simulink model "gm_uz_pmsm_model_6LUT_pd"  (R2023a)
settings: Solver=FixedStepAuto  StartTime=0.0  StopTime=0.05  RelTol=1e-3
PreLoadFcn:
  | uz_pmsm_model_init_parameter
PostLoadFcn:
  | % Import the data from Excel for a lookup table
  | FluxMapData = readtable('C:\Users\Philipp\ultrazohm\ultrazohm_sw\ip_cores\uz_pmsm_model\FluxMapData_2023-05-26_13-07-57.csv');
  | % Row indices for lookup table
  | d_current_in_d_axis = FluxMapData(8:27,1:end);
  | % Column indices for lookup table
  | q_current_in_d_axis = FluxMapData(29:48,1:end);
  | % Output values for lookup table
  | d_Flux_d_axis = FluxMapData(50:69,1:end);
undefined symbols (not defined in the file or in its folder): d_current_d_Flux, d_current_q_Flux, entkopplung_dynamic, entkopplung_linear, entkopplung_static, Flux_d, Flux_q, friction_coefficient, inertia, k_i_d, k_p_d, k_p_q, Ki_Bo_d, Ki_Bo_q, Kp_Bo_d, Kp_Bo_q, L_d, L_q, Ldd, Ldq, Lqd, Lqq, parameter_nachfuerung, polepair, praediktion_entkopplung_nonlinear, psi_pm, q_current_d_Flux, q_current_q_Flux, R_1, simulate_mechanical, simulate_nonlinear_modell, simulate_open_loop, static_friction_torque, tau_sum, ts, ts_regler
libraries: hdlmdlgenlib x5, slpidlib x4
(part 2 of 2)

== system gm_uz_pmsm_model_6LUT_pd/Current_Controller/Psi_d_q ==
  I_d_set : Inport
  I_d : Inport  Port=2
  I_q_set : Inport  Port=3
  I_q : Inport  Port=4
  Flux_d Lookup Table : Lookup_n-D  BreakpointsForDimension1=d_current_d_Flux  BreakpointsForDimension2=q_current_d_Flux  BreakpointsForDimension3=[5, 7]  Table=Flux_d  InternalRulePriority=Speed  RndMeth=Simplest
      settings: InputPortMap=u0,u1
  Flux_d Lookup Table1 : Lookup_n-D  BreakpointsForDimension1=d_current_d_Flux  BreakpointsForDimension2=q_current_d_Flux  BreakpointsForDimension3=[5, 7]  Table=Flux_d  InternalRulePriority=Speed  RndMeth=Simplest
      settings: InputPortMap=u0,u1
  Flux_q Lookup Table1 : Lookup_n-D  BreakpointsForDimension1=d_current_q_Flux  BreakpointsForDimension2=q_current_q_Flux  BreakpointsForDimension3=[5, 7]  Table=Flux_q  InternalRulePriority=Speed  RndMeth=Simplest
      settings: InputPortMap=u0,u1
  Flux_q Lookup Table2 : Lookup_n-D  BreakpointsForDimension1=d_current_q_Flux  BreakpointsForDimension2=q_current_q_Flux  BreakpointsForDimension3=[5, 7]  Table=Flux_q  InternalRulePriority=Speed  RndMeth=Simplest
      settings: InputPortMap=u0,u1
  psi_d_set : Outport
  psi_q_set : Outport  Port=2
  psi_d_LUT : Outport  Port=3
  psi_q_LUT : Outport  Port=4
  wires:
  Flux_q Lookup Table1/1 -> psi_q_LUT/1  "psi_q_LUT"
  Flux_d Lookup Table/1 -> psi_d_LUT/1  "psi_d_LUT"
  Flux_q Lookup Table2/1 -> psi_q_set/1  "psi_q_set"
  Flux_d Lookup Table1/1 -> psi_d_set/1  "psi_d_set"
  I_q_set/1 -> Flux_q Lookup Table2/2
  I_d_set/1 -> Flux_d Lookup Table1/1
  I_q/1 -> Flux_d Lookup Table/2, Flux_d Lookup Table1/2, Flux_q Lookup Table1/2
  I_d/1 -> Flux_d Lookup Table/1, Flux_q Lookup Table1/1, Flux_q Lookup Table2/1

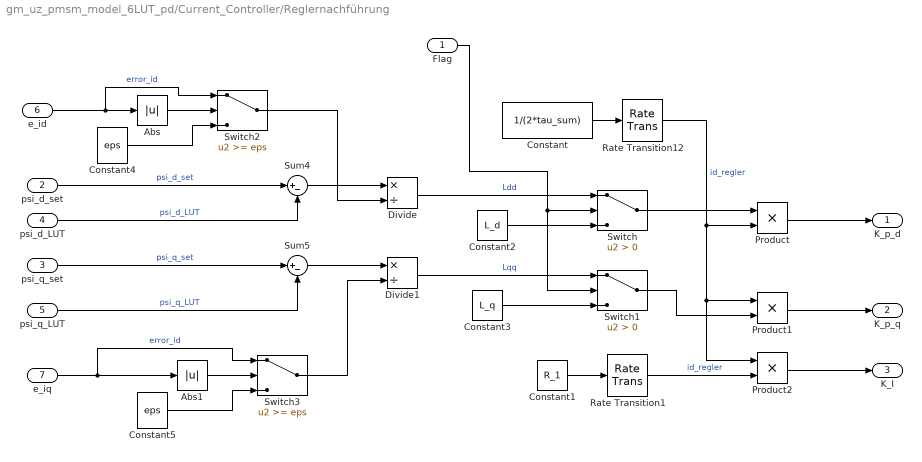
== system gm_uz_pmsm_model_6LUT_pd/Current_Controller/Reglernachführung ==
  Flag : Inport
  psi_d_set : Inport  Port=2
  psi_q_set : Inport  Port=3
  psi_d_LUT : Inport  Port=4
  psi_q_LUT : Inport  Port=5
  e_id : Inport  Port=6
  e_iq : Inport  Port=7
  Abs : Abs  SaturateOnIntegerOverflow=off
  Abs1 : Abs  SaturateOnIntegerOverflow=off
  Constant : Constant  Value=1/(2*tau_sum)
  Constant1 : Constant  Value=R_1
  Constant2 : Constant  Value=L_d
  Constant3 : Constant  Value=L_q
  Constant4 : Constant  Value=eps  SampleTime=ts_regler
  Constant5 : Constant  Value=eps  SampleTime=ts_regler
  Divide : Product  Inputs=*/
  Divide1 : Product  Inputs=*/
  Product : Product
  Product1 : Product
  Product2 : Product
  Rate Transition1 : RateTransition  OutPortSampleTime=ts_regler
  Rate Transition12 : RateTransition  OutPortSampleTime=ts_regler
  Sum4 : Sum  Inputs=|+-
  Sum5 : Sum  Inputs=|+-
  Switch : Switch  Criteria=u2 > Threshold  SaturateOnIntegerOverflow=off  InputSameDT=off
  Switch1 : Switch  Criteria=u2 > Threshold  SaturateOnIntegerOverflow=off  InputSameDT=off
  Switch2 : Switch  Threshold=eps  SaturateOnIntegerOverflow=off  InputSameDT=off
  Switch3 : Switch  Threshold=eps  SaturateOnIntegerOverflow=off  InputSameDT=off
  K_p_d : Outport
  K_p_q : Outport  Port=2
  K_I : Outport  Port=3
  wires:
  Constant5/1 -> Switch3/3
  Abs1/1 -> Switch3/2
  Switch3/1 -> Divide1/2
  e_iq/1 -> Abs1/1, Switch3/1  "error_id"
  Switch2/1 -> Divide/2
  Abs/1 -> Switch2/2
  Constant4/1 -> Switch2/3
  e_id/1 -> Abs/1, Switch2/1  "error_id"
  Divide1/1 -> Switch1/1  "Lqq"
  Divide/1 -> Switch/1  "Ldd"
  psi_q_set/1 -> Sum5/1  "psi_q_set"
  psi_d_set/1 -> Sum4/1  "psi_d_set"
  psi_d_LUT/1 -> Sum4/2  "psi_d_LUT"
  Sum5/1 -> Divide1/1
  psi_q_LUT/1 -> Sum5/2  "psi_q_LUT"
  Sum4/1 -> Divide/1
  Switch1/1 -> Product1/2
  Constant3/1 -> Switch1/3
  Switch/1 -> Product/1
  Constant2/1 -> Switch/3
  Flag/1 -> Switch1/2, Switch/2
  Rate Transition1/1 -> Product2/2  "id_regler"
  Rate Transition12/1 -> Product/2, Product1/1, Product2/1  "id_regler"
  Constant1/1 -> Rate Transition1/1
  Product2/1 -> K_I/1
  Product1/1 -> K_p_q/1
  Product/1 -> K_p_d/1
  Constant/1 -> Rate Transition12/1

== system gm_uz_pmsm_model_6LUT_pd/FOC_controller1/Psi_d_q ==
  I_d_set : Inport
  I_d : Inport  Port=2
  I_q_set : Inport  Port=3
  I_q : Inport  Port=4
  Flux_d Lookup Table : Lookup_n-D  BreakpointsForDimension1=d_current_d_Flux  BreakpointsForDimension2=q_current_d_Flux  BreakpointsForDimension3=[5, 7]  Table=Flux_d  InternalRulePriority=Speed  RndMeth=Simplest
      settings: InputPortMap=u0,u1
  Flux_d Lookup Table1 : Lookup_n-D  BreakpointsForDimension1=d_current_d_Flux  BreakpointsForDimension2=q_current_d_Flux  BreakpointsForDimension3=[5, 7]  Table=Flux_d  InternalRulePriority=Speed  RndMeth=Simplest
      settings: InputPortMap=u0,u1
  Flux_q Lookup Table1 : Lookup_n-D  BreakpointsForDimension1=d_current_q_Flux  BreakpointsForDimension2=q_current_q_Flux  BreakpointsForDimension3=[5, 7]  Table=Flux_q  InternalRulePriority=Speed  RndMeth=Simplest
      settings: InputPortMap=u0,u1
  Flux_q Lookup Table2 : Lookup_n-D  BreakpointsForDimension1=d_current_q_Flux  BreakpointsForDimension2=q_current_q_Flux  BreakpointsForDimension3=[5, 7]  Table=Flux_q  InternalRulePriority=Speed  RndMeth=Simplest
      settings: InputPortMap=u0,u1
  psi_d_set : Outport
  psi_q_set : Outport  Port=2
  psi_d_LUT : Outport  Port=3
  psi_q_LUT : Outport  Port=4
  wires:
  Flux_q Lookup Table1/1 -> psi_q_LUT/1  "psi_q_LUT"
  Flux_d Lookup Table/1 -> psi_d_LUT/1  "psi_d_LUT"
  Flux_q Lookup Table2/1 -> psi_q_set/1  "psi_q_set"
  Flux_d Lookup Table1/1 -> psi_d_set/1  "psi_d_set"
  I_q_set/1 -> Flux_q Lookup Table2/2
  I_d_set/1 -> Flux_d Lookup Table1/1
  I_q/1 -> Flux_d Lookup Table/2, Flux_d Lookup Table1/2, Flux_q Lookup Table1/2
  I_d/1 -> Flux_d Lookup Table/1, Flux_q Lookup Table1/1, Flux_q Lookup Table2/1

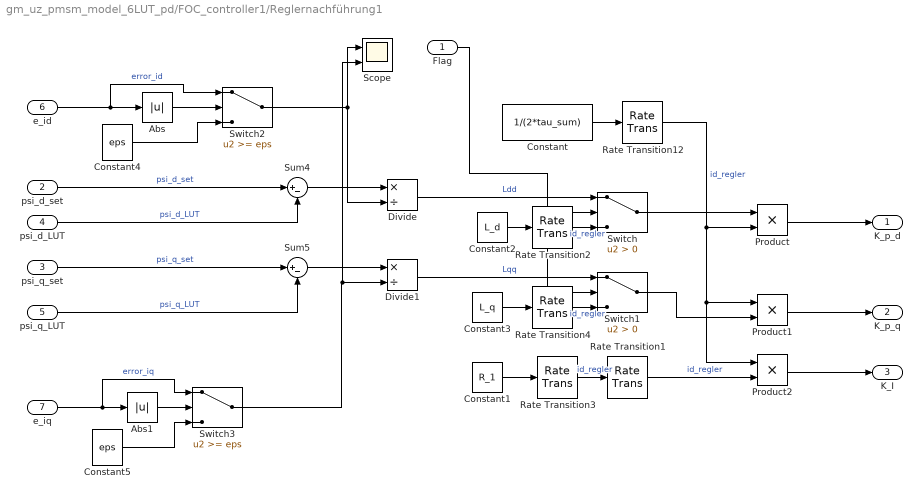
== system gm_uz_pmsm_model_6LUT_pd/FOC_controller1/Reglernachführung1 ==
  Flag : Inport
  psi_d_set : Inport  Port=2
  psi_q_set : Inport  Port=3
  psi_d_LUT : Inport  Port=4
  psi_q_LUT : Inport  Port=5
  e_id : Inport  Port=6
  e_iq : Inport  Port=7
  Abs : Abs  SaturateOnIntegerOverflow=off
  Abs1 : Abs  SaturateOnIntegerOverflow=off
  Constant : Constant  Value=1/(2*tau_sum)
  Constant1 : Constant  Value=R_1
  Constant2 : Constant  Value=L_d
  Constant3 : Constant  Value=L_q
  Constant4 : Constant  Value=eps  SampleTime=ts_regler
  Constant5 : Constant  Value=eps  SampleTime=ts_regler
  Divide : Product  Inputs=*/
  Divide1 : Product  Inputs=*/
  Product : Product
  Product1 : Product
  Product2 : Product
  Rate Transition{1..4,12} (5 alike) : RateTransition  OutPortSampleTime=ts_regler
  Scope : Scope  NumInputPorts=2
  Sum4 : Sum  Inputs=|+-
  Sum5 : Sum  Inputs=|+-
  Switch : Switch  Criteria=u2 > Threshold  SaturateOnIntegerOverflow=off  InputSameDT=off
  Switch1 : Switch  Criteria=u2 > Threshold  SaturateOnIntegerOverflow=off  InputSameDT=off
  Switch2 : Switch  Threshold=eps  SaturateOnIntegerOverflow=off  InputSameDT=off
  Switch3 : Switch  Threshold=eps  SaturateOnIntegerOverflow=off  InputSameDT=off
  K_p_d : Outport
  K_p_q : Outport  Port=2
  K_I : Outport  Port=3
  wires:
  Rate Transition4/1 -> Switch1/3  "id_regler"
  Rate Transition3/1 -> Rate Transition1/1  "id_regler"
  Rate Transition2/1 -> Switch/3  "id_regler"
  Switch3/1 -> Divide1/2, Scope/2
  Constant5/1 -> Switch3/3
  Switch2/1 -> Divide/2, Scope/1
  Constant4/1 -> Switch2/3
  Abs/1 -> Switch2/2
  Divide1/1 -> Switch1/1  "Lqq"
  Divide/1 -> Switch/1  "Ldd"
  psi_q_set/1 -> Sum5/1  "psi_q_set"
  psi_d_set/1 -> Sum4/1  "psi_d_set"
  psi_d_LUT/1 -> Sum4/2  "psi_d_LUT"
  Sum5/1 -> Divide1/1
  psi_q_LUT/1 -> Sum5/2  "psi_q_LUT"
  Abs1/1 -> Switch3/2
  Sum4/1 -> Divide/1
  e_iq/1 -> Abs1/1, Switch3/1  "error_iq"
  e_id/1 -> Abs/1, Switch2/1  "error_id"
  Switch1/1 -> Product1/2
  Constant3/1 -> Rate Transition4/1
  Switch/1 -> Product/1
  Constant2/1 -> Rate Transition2/1
  Flag/1 -> Switch1/2, Switch/2
  Rate Transition1/1 -> Product2/2  "id_regler"
  Rate Transition12/1 -> Product/2, Product1/1, Product2/1  "id_regler"
  Constant1/1 -> Rate Transition3/1
  Product2/1 -> K_I/1
  Product1/1 -> K_p_q/1
  Product/1 -> K_p_d/1
  Constant/1 -> Rate Transition12/1

== system gm_uz_pmsm_model_6LUT_pd/FOC_controller1/decoupling2 ==
  i_d : Inport
  i_q : Inport  Port=2
  omega_m : Inport  Port=3
  Flux_d Lookup Table : Lookup_n-D  BreakpointsForDimension1=d_current_d_Flux  BreakpointsForDimension2=q_current_d_Flux  BreakpointsForDimension3=[5, 7]  Table=Flux_d  InternalRulePriority=Speed  RndMeth=Simplest
      settings: InputPortMap=u0,u1
  Flux_q Lookup Table1 : Lookup_n-D  BreakpointsForDimension1=d_current_q_Flux  BreakpointsForDimension2=q_current_q_Flux  BreakpointsForDimension3=[5, 7]  Table=Flux_q  InternalRulePriority=Speed  RndMeth=Simplest
      settings: InputPortMap=u0,u1
  Gain2 : Gain  Gain=polepair
  Product : Product
  Product1 : Product
  Scope : Scope  NumInputPorts=2
  u_d : Outport
  u_q : Outport  Port=2
  wires:
  omega_m/1 -> Gain2/1
  Flux_q Lookup Table1/1 -> Product1/1
  i_q/1 -> Flux_d Lookup Table/2, Flux_q Lookup Table1/2
  Product/1 -> u_d/1, Scope/2
  i_d/1 -> Flux_d Lookup Table/1, Flux_q Lookup Table1/1
  Product1/1 -> u_q/1, Scope/1
  Gain2/1 -> Product/2, Product1/2
  Flux_d Lookup Table/1 -> Product/1

== system gm_uz_pmsm_model_6LUT_pd/pmsm/Subsystem ==
  in : Inport
  reset : Inport  Port=2
  Delay1 : Delay  DelayLength=1  ExternalReset=Level
      settings: InputPortMap=u0,r5
  Gain7 : Gain  Gain=ts  OutDataTypeStr=double
  Sum5 : Sum  Inputs=|++  OutDataTypeStr=double
  outt : Outport
  wires:
  Sum5/1 -> Delay1/1
  Gain7/1 -> Sum5/1
  Delay1/1 -> Sum5/2, outt/1
  reset/1 -> Delay1/2
  in/1 -> Gain7/1

== system gm_uz_pmsm_model_6LUT_pd/pmsm/Subsystem1 ==
  in : Inport
  reset : Inport  Port=2
  Delay1 : Delay  DelayLength=1  ExternalReset=Level
      settings: InputPortMap=u0,r5
  Gain7 : Gain  Gain=ts  OutDataTypeStr=double
  Sum5 : Sum  Inputs=|++  OutDataTypeStr=double
  outt : Outport
  wires:
  Sum5/1 -> Delay1/1
  Gain7/1 -> Sum5/1
  Delay1/1 -> Sum5/2, outt/1
  reset/1 -> Delay1/2
  in/1 -> Gain7/1

== system gm_uz_pmsm_model_6LUT_pd/uz_pmsm_model_6LUT/Abs ==
  In1 : Inport
  Abs : Abs  SampleTime=1e-08  OutDataTypeStr=single  SaturateOnIntegerOverflow=off
  Out1 : Outport
  wires:
  In1/1 -> Abs/1
  Abs/1 -> Out1/1

== system gm_uz_pmsm_model_6LUT_pd/uz_pmsm_model_6LUT/Divide ==
  In1 : Inport
  In2 : Inport  Port=2
  Divide : Product  Inputs=**  OutDataTypeStr=single  SampleTime=1e-08
  Divide_pd1 : Delay  DelayLength=6
  Out1 : Outport
  wires:
  In1/1 -> Divide/1
  In2/1 -> Divide/2
  Divide/1 -> Divide_pd1/1
  Divide_pd1/1 -> Out1/1

== system gm_uz_pmsm_model_6LUT_pd/uz_pmsm_model_6LUT/Divide1 ==
  In1 : Inport
  In2 : Inport  Port=2
  Divide1 : Product  Inputs=*/  OutDataTypeStr=single  SampleTime=1e-08
  Divide1_pd1 : Delay  DelayLength=17
  Out1 : Outport
  wires:
  In1/1 -> Divide1/1
  In2/1 -> Divide1/2
  Divide1/1 -> Divide1_pd1/1
  Divide1_pd1/1 -> Out1/1

== system gm_uz_pmsm_model_6LUT_pd/uz_pmsm_model_6LUT/Divide_recip ==
  In1 : Inport
  Divide_recip : Math  Operator=reciprocal  SampleTime=1e-08
  Divide_recip_pd1 : Delay  DelayLength=16
  Out1 : Outport
  wires:
  In1/1 -> Divide_recip/1
  Divide_recip/1 -> Divide_recip_pd1/1
  Divide_recip_pd1/1 -> Out1/1

== system gm_uz_pmsm_model_6LUT_pd/uz_pmsm_model_6LUT/Factor ==
  In1 : Inport
  In2 : Inport  Port=2
  Factor : Product  Inputs=**  OutDataTypeStr=single  SampleTime=1e-08
  Factor_pd1 : Delay  DelayLength=6
  Out1 : Outport
  wires:
  In1/1 -> Factor/1
  In2/1 -> Factor/2
  Factor/1 -> Factor_pd1/1
  Factor_pd1/1 -> Out1/1

== system gm_uz_pmsm_model_6LUT_pd/uz_pmsm_model_6LUT/Flux_d Lookup Table ==
  In1 : Inport
  In2 : Inport  Port=2
  Flux_d Lookup Table : Lookup_n-D  BreakpointsForDimension1=d_current_q_Flux  BreakpointsForDimension2=q_current_q_Flux  BreakpointsForDimension3=[5, 7]  Table=Flux_d  ExtrapMethod=Clip  UseLastTableValue=on  InternalRulePriority=Speed  OutDataTypeStr=Inherit: Inherit from 'Table data'  RndMeth=Simplest
      settings: InputPortMap=u0,u1
  Flux_d Lookup Table_pd1 : Delay  DelayLength=53
  Out1 : Outport
  wires:
  Flux_d Lookup Table_pd1/1 -> Out1/1
  Flux_d Lookup Table/1 -> Flux_d Lookup Table_pd1/1
  In1/1 -> Flux_d Lookup Table/1
  In2/1 -> Flux_d Lookup Table/2

== system gm_uz_pmsm_model_6LUT_pd/uz_pmsm_model_6LUT/Flux_q Lookup Table ==
  In1 : Inport
  In2 : Inport  Port=2
  Flux_q Lookup Table : Lookup_n-D  BreakpointsForDimension1=d_current_q_Flux  BreakpointsForDimension2=q_current_q_Flux  BreakpointsForDimension3=[5, 7]  Table=Flux_q  ExtrapMethod=Clip  UseLastTableValue=on  InternalRulePriority=Speed  OutDataTypeStr=Inherit: Inherit from 'Table data'  RndMeth=Simplest
      settings: InputPortMap=u0,u1
  Flux_q Lookup Table_pd1 : Delay  DelayLength=53
  Out1 : Outport
  wires:
  Flux_q Lookup Table_pd1/1 -> Out1/1
  Flux_q Lookup Table/1 -> Flux_q Lookup Table_pd1/1
  In1/1 -> Flux_q Lookup Table/1
  In2/1 -> Flux_q Lookup Table/2

== system gm_uz_pmsm_model_6LUT_pd/uz_pmsm_model_6LUT/Gain ==
  In1 : Inport
  In2 : Inport  Port=2
  Gain : Product  Inputs=**  OutDataTypeStr=single  SampleTime=1e-08
  Gain_pd1 : Delay  DelayLength=6
  Out1 : Outport
  wires:
  In1/1 -> Gain/1
  In2/1 -> Gain/2
  Gain/1 -> Gain_pd1/1
  Gain_pd1/1 -> Out1/1

== system gm_uz_pmsm_model_6LUT_pd/uz_pmsm_model_6LUT/Gain7 ==
  In1 : Inport
  In2 : Inport  Port=2
  Gain7 : Product  Inputs=**  OutDataTypeStr=single  SampleTime=1e-08
  Gain7_pd1 : Delay  DelayLength=6
  Out1 : Outport
  wires:
  In1/1 -> Gain7/1
  In2/1 -> Gain7/2
  Gain7/1 -> Gain7_pd1/1
  Gain7_pd1/1 -> Out1/1

== system gm_uz_pmsm_model_6LUT_pd/uz_pmsm_model_6LUT/Gain71 ==
  In1 : Inport
  In2 : Inport  Port=2
  Gain71 : Product  Inputs=**  OutDataTypeStr=single  SampleTime=1e-08
  Gain71_pd1 : Delay  DelayLength=6
  Out1 : Outport
  wires:
  In1/1 -> Gain71/1
  In2/1 -> Gain71/2
  Gain71/1 -> Gain71_pd1/1
  Gain71_pd1/1 -> Out1/1

== system gm_uz_pmsm_model_6LUT_pd/uz_pmsm_model_6LUT/Ldd Lookup Table ==
  In1 : Inport
  In2 : Inport  Port=2
  Ldd Lookup Table : Lookup_n-D  BreakpointsForDimension1=d_current_q_Flux  BreakpointsForDimension2=q_current_q_Flux  BreakpointsForDimension3=[5, 7]  Table=Ldd  ExtrapMethod=Clip  UseLastTableValue=on  InternalRulePriority=Speed  OutDataTypeStr=Inherit: Inherit from 'Table data'  RndMeth=Simplest
      settings: InputPortMap=u0,u1
  Ldd Lookup Table_pd1 : Delay  DelayLength=53
  Out1 : Outport
  wires:
  In2/1 -> Ldd Lookup Table/2
  In1/1 -> Ldd Lookup Table/1
  Ldd Lookup Table/1 -> Ldd Lookup Table_pd1/1
  Ldd Lookup Table_pd1/1 -> Out1/1

== system gm_uz_pmsm_model_6LUT_pd/uz_pmsm_model_6LUT/Ldq Lookup Table2 ==
  In1 : Inport
  In2 : Inport  Port=2
  Ldq Lookup Table2 : Lookup_n-D  BreakpointsForDimension1=d_current_q_Flux  BreakpointsForDimension2=q_current_q_Flux  BreakpointsForDimension3=[5, 7]  Table=Ldq  ExtrapMethod=Clip  UseLastTableValue=on  InternalRulePriority=Speed  OutDataTypeStr=Inherit: Inherit from 'Table data'  RndMeth=Simplest
      settings: InputPortMap=u0,u1
  Ldq Lookup Table2_pd1 : Delay  DelayLength=53
  Out1 : Outport
  wires:
  Ldq Lookup Table2_pd1/1 -> Out1/1
  Ldq Lookup Table2/1 -> Ldq Lookup Table2_pd1/1
  In2/1 -> Ldq Lookup Table2/2
  In1/1 -> Ldq Lookup Table2/1

== system gm_uz_pmsm_model_6LUT_pd/uz_pmsm_model_6LUT/Lqd Lookup Table1 ==
  In1 : Inport
  In2 : Inport  Port=2
  Lqd Lookup Table1 : Lookup_n-D  BreakpointsForDimension1=d_current_q_Flux  BreakpointsForDimension2=q_current_q_Flux  BreakpointsForDimension3=[5, 7]  Table=Lqd  ExtrapMethod=Clip  UseLastTableValue=on  InternalRulePriority=Speed  OutDataTypeStr=Inherit: Inherit from 'Table data'  RndMeth=Simplest
      settings: InputPortMap=u0,u1
  Lqd Lookup Table1_pd1 : Delay  DelayLength=53
  Out1 : Outport
  wires:
  Lqd Lookup Table1_pd1/1 -> Out1/1
  Lqd Lookup Table1/1 -> Lqd Lookup Table1_pd1/1
  In2/1 -> Lqd Lookup Table1/2
  In1/1 -> Lqd Lookup Table1/1

== system gm_uz_pmsm_model_6LUT_pd/uz_pmsm_model_6LUT/Lqq Lookup Table ==
  In1 : Inport
  In2 : Inport  Port=2
  Lqq Lookup Table : Lookup_n-D  BreakpointsForDimension1=d_current_q_Flux  BreakpointsForDimension2=q_current_q_Flux  BreakpointsForDimension3=[5, 7]  Table=Lqq  ExtrapMethod=Clip  UseLastTableValue=on  InternalRulePriority=Speed  OutDataTypeStr=Inherit: Inherit from 'Table data'  RndMeth=Simplest
      settings: InputPortMap=u0,u1
  Lqq Lookup Table_pd1 : Delay  DelayLength=53
  Out1 : Outport
  wires:
  In1/1 -> Lqq Lookup Table/1
  Lqq Lookup Table_pd1/1 -> Out1/1
  In2/1 -> Lqq Lookup Table/2
  Lqq Lookup Table/1 -> Lqq Lookup Table_pd1/1

== system gm_uz_pmsm_model_6LUT_pd/uz_pmsm_model_6LUT/Product11 ==
  In1 : Inport
  In2 : Inport  Port=2
  Product11 : Product  Inputs=**  OutDataTypeStr=single  SampleTime=1e-08
  Product11_pd1 : Delay  DelayLength=6
  Out1 : Outport
  wires:
  In1/1 -> Product11/1
  In2/1 -> Product11/2
  Product11/1 -> Product11_pd1/1
  Product11_pd1/1 -> Out1/1

== system gm_uz_pmsm_model_6LUT_pd/uz_pmsm_model_6LUT/Product111 ==
  In1 : Inport
  In2 : Inport  Port=2
  Product111 : Product  Inputs=**  OutDataTypeStr=single  SampleTime=1e-08
  Product111_pd1 : Delay  DelayLength=6
  Out1 : Outport
  wires:
  In1/1 -> Product111/1
  In2/1 -> Product111/2
  Product111/1 -> Product111_pd1/1
  Product111_pd1/1 -> Out1/1

== system gm_uz_pmsm_model_6LUT_pd/uz_pmsm_model_6LUT/Product12 ==
  In1 : Inport
  In2 : Inport  Port=2
  Product12 : Product  Inputs=**  OutDataTypeStr=single  SampleTime=1e-08
  Product12_pd1 : Delay  DelayLength=6
  Out1 : Outport
  wires:
  In1/1 -> Product12/1
  In2/1 -> Product12/2
  Product12/1 -> Product12_pd1/1
  Product12_pd1/1 -> Out1/1

== system gm_uz_pmsm_model_6LUT_pd/uz_pmsm_model_6LUT/Product121 ==
  In1 : Inport
  In2 : Inport  Port=2
  Product121 : Product  Inputs=**  OutDataTypeStr=single  SampleTime=1e-08
  Product121_pd1 : Delay  DelayLength=6
  Out1 : Outport
  wires:
  In1/1 -> Product121/1
  In2/1 -> Product121/2
  Product121/1 -> Product121_pd1/1
  Product121_pd1/1 -> Out1/1

== system gm_uz_pmsm_model_6LUT_pd/uz_pmsm_model_6LUT/Product13 ==
  In1 : Inport
  In2 : Inport  Port=2
  Product13 : Product  Inputs=**  OutDataTypeStr=single  SampleTime=1e-08
  Product13_pd1 : Delay  DelayLength=6
  Out1 : Outport
  wires:
  In1/1 -> Product13/1
  In2/1 -> Product13/2
  Product13/1 -> Product13_pd1/1
  Product13_pd1/1 -> Out1/1

== system gm_uz_pmsm_model_6LUT_pd/uz_pmsm_model_6LUT/Product2 ==
  In1 : Inport
  In2 : Inport  Port=2
  Product2 : Product  Inputs=**  OutDataTypeStr=single  SampleTime=1e-08
  Product2_pd1 : Delay  DelayLength=6
  Out1 : Outport
  wires:
  In1/1 -> Product2/1
  In2/1 -> Product2/2
  Product2/1 -> Product2_pd1/1
  Product2_pd1/1 -> Out1/1

== system gm_uz_pmsm_model_6LUT_pd/uz_pmsm_model_6LUT/Product21 ==
  In1 : Inport
  In2 : Inport  Port=2
  Product21 : Product  Inputs=**  OutDataTypeStr=single  SampleTime=1e-08
  Product21_pd1 : Delay  DelayLength=6
  Out1 : Outport
  wires:
  In1/1 -> Product21/1
  In2/1 -> Product21/2
  Product21/1 -> Product21_pd1/1
  Product21_pd1/1 -> Out1/1

== system gm_uz_pmsm_model_6LUT_pd/uz_pmsm_model_6LUT/Product3 ==
  In1 : Inport
  In2 : Inport  Port=2
  Product3 : Product  Inputs=**  OutDataTypeStr=single  SampleTime=1e-08
  Product3_pd1 : Delay  DelayLength=6
  Out1 : Outport
  wires:
  In1/1 -> Product3/1
  In2/1 -> Product3/2
  Product3/1 -> Product3_pd1/1
  Product3_pd1/1 -> Out1/1

== system gm_uz_pmsm_model_6LUT_pd/uz_pmsm_model_6LUT/Product31 ==
  In1 : Inport
  In2 : Inport  Port=2
  Product31 : Product  Inputs=**  OutDataTypeStr=single  SampleTime=1e-08
  Product31_pd1 : Delay  DelayLength=6
  Out1 : Outport
  wires:
  In1/1 -> Product31/1
  In2/1 -> Product31/2
  Product31/1 -> Product31_pd1/1
  Product31_pd1/1 -> Out1/1

== system gm_uz_pmsm_model_6LUT_pd/uz_pmsm_model_6LUT/Product4 ==
  In1 : Inport
  In2 : Inport  Port=2
  Product4 : Product  Inputs=**  OutDataTypeStr=single  SampleTime=1e-08
  Product4_pd1 : Delay  DelayLength=6
  Out1 : Outport
  wires:
  In1/1 -> Product4/1
  In2/1 -> Product4/2
  Product4/1 -> Product4_pd1/1
  Product4_pd1/1 -> Out1/1

== system gm_uz_pmsm_model_6LUT_pd/uz_pmsm_model_6LUT/Product41 ==
  In1 : Inport
  In2 : Inport  Port=2
  Product41 : Product  Inputs=**  OutDataTypeStr=single  SampleTime=1e-08
  Product41_pd1 : Delay  DelayLength=6
  Out1 : Outport
  wires:
  In1/1 -> Product41/1
  In2/1 -> Product41/2
  Product41/1 -> Product41_pd1/1
  Product41_pd1/1 -> Out1/1

== system gm_uz_pmsm_model_6LUT_pd/uz_pmsm_model_6LUT/Product9 ==
  In1 : Inport
  In2 : Inport  Port=2
  Product9 : Product  Inputs=**  OutDataTypeStr=single  SampleTime=1e-08
  Product9_pd1 : Delay  DelayLength=6
  Out1 : Outport
  wires:
  In1/1 -> Product9/1
  In2/1 -> Product9/2
  Product9/1 -> Product9_pd1/1
  Product9_pd1/1 -> Out1/1

== system gm_uz_pmsm_model_6LUT_pd/uz_pmsm_model_6LUT/Product91 ==
  In1 : Inport
  In2 : Inport  Port=2
  Product91 : Product  Inputs=**  OutDataTypeStr=single  SampleTime=1e-08
  Product91_pd1 : Delay  DelayLength=6
  Out1 : Outport
  wires:
  In1/1 -> Product91/1
  In2/1 -> Product91/2
  Product91/1 -> Product91_pd1/1
  Product91_pd1/1 -> Out1/1

== system gm_uz_pmsm_model_6LUT_pd/uz_pmsm_model_6LUT/Sign1 ==
  In1 : Inport
  Sign1 : Signum  SampleTime=1e-08
  Out1 : Outport
  wires:
  In1/1 -> Sign1/1
  Sign1/1 -> Out1/1

== system gm_uz_pmsm_model_6LUT_pd/uz_pmsm_model_6LUT/Sum ==
  In1 : Inport
  In2 : Inport  Port=2
  Sum : Sum  Inputs=+-  OutDataTypeStr=single  SampleTime=1e-08
  Sum_pd1 : Delay  DelayLength=6
  Out1 : Outport
  wires:
  In1/1 -> Sum/1
  In2/1 -> Sum/2
  Sum/1 -> Sum_pd1/1
  Sum_pd1/1 -> Out1/1

== system gm_uz_pmsm_model_6LUT_pd/uz_pmsm_model_6LUT/Sum1 ==
  In1 : Inport
  In2 : Inport  Port=2
  Sum1 : Sum  Inputs=+-  OutDataTypeStr=single  SampleTime=1e-08
  Sum1_pd1 : Delay  DelayLength=6
  Out1 : Outport
  wires:
  In1/1 -> Sum1/1
  In2/1 -> Sum1/2
  Sum1/1 -> Sum1_pd1/1
  Sum1_pd1/1 -> Out1/1

== system gm_uz_pmsm_model_6LUT_pd/uz_pmsm_model_6LUT/Sum3 ==
  In1 : Inport
  In2 : Inport  Port=2
  Sum3 : Sum  OutDataTypeStr=single  SampleTime=1e-08
  Sum3_pd1 : Delay  DelayLength=6
  Out1 : Outport
  wires:
  In1/1 -> Sum3/1
  In2/1 -> Sum3/2
  Sum3/1 -> Sum3_pd1/1
  Sum3_pd1/1 -> Out1/1

== system gm_uz_pmsm_model_6LUT_pd/uz_pmsm_model_6LUT/Sum31 ==
  In1 : Inport
  In2 : Inport  Port=2
  Sum31 : Sum  Inputs=+-  OutDataTypeStr=single  SampleTime=1e-08
  Sum31_pd1 : Delay  DelayLength=6
  Out1 : Outport
  wires:
  In1/1 -> Sum31/1
  In2/1 -> Sum31/2
  Sum31/1 -> Sum31_pd1/1
  Sum31_pd1/1 -> Out1/1

== system gm_uz_pmsm_model_6LUT_pd/uz_pmsm_model_6LUT/Sum3_stage2 ==
  In1 : Inport
  In2 : Inport  Port=2
  Sum3_stage2 : Sum  Inputs=+-  OutDataTypeStr=single  SampleTime=1e-08
  Sum3_stage2_pd1 : Delay  DelayLength=6
  Out1 : Outport
  wires:
  In1/1 -> Sum3_stage2/1
  In2/1 -> Sum3_stage2/2
  Sum3_stage2/1 -> Sum3_stage2_pd1/1
  Sum3_stage2_pd1/1 -> Out1/1

== system gm_uz_pmsm_model_6LUT_pd/uz_pmsm_model_6LUT/Sum3_stage3 ==
  In1 : Inport
  In2 : Inport  Port=2
  Sum3_stage3 : Sum  Inputs=+-  OutDataTypeStr=single  SampleTime=1e-08
  Sum3_stage3_pd1 : Delay  DelayLength=6
  Out1 : Outport
  wires:
  In1/1 -> Sum3_stage3/1
  In2/1 -> Sum3_stage3/2
  Sum3_stage3/1 -> Sum3_stage3_pd1/1
  Sum3_stage3_pd1/1 -> Out1/1

== system gm_uz_pmsm_model_6LUT_pd/uz_pmsm_model_6LUT/Sum3_stage4 ==
  In1 : Inport
  In2 : Inport  Port=2
  Sum3_stage4 : Sum  OutDataTypeStr=single  SampleTime=1e-08
  Sum3_stage4_pd1 : Delay  DelayLength=6
  Out1 : Outport
  wires:
  In1/1 -> Sum3_stage4/1
  In2/1 -> Sum3_stage4/2
  Sum3_stage4/1 -> Sum3_stage4_pd1/1
  Sum3_stage4_pd1/1 -> Out1/1

== system gm_uz_pmsm_model_6LUT_pd/uz_pmsm_model_6LUT/Sum4_stage2 ==
  In1 : Inport
  In2 : Inport  Port=2
  Sum4_stage2 : Sum  Inputs=+-  OutDataTypeStr=single  SampleTime=1e-08
  Sum4_stage2_pd1 : Delay  DelayLength=6
  Out1 : Outport
  wires:
  In1/1 -> Sum4_stage2/1
  In2/1 -> Sum4_stage2/2
  Sum4_stage2/1 -> Sum4_stage2_pd1/1
  Sum4_stage2_pd1/1 -> Out1/1

== system gm_uz_pmsm_model_6LUT_pd/uz_pmsm_model_6LUT/Sum4_stage3 ==
  In1 : Inport
  In2 : Inport  Port=2
  Sum4_stage3 : Sum  Inputs=+-  OutDataTypeStr=single  SampleTime=1e-08
  Sum4_stage3_pd1 : Delay  DelayLength=6
  Out1 : Outport
  wires:
  In1/1 -> Sum4_stage3/1
  In2/1 -> Sum4_stage3/2
  Sum4_stage3/1 -> Sum4_stage3_pd1/1
  Sum4_stage3_pd1/1 -> Out1/1

== system gm_uz_pmsm_model_6LUT_pd/uz_pmsm_model_6LUT/Sum4_stage4 ==
  In1 : Inport
  In2 : Inport  Port=2
  Sum4_stage4 : Sum  Inputs=+-  OutDataTypeStr=single  SampleTime=1e-08
  Sum4_stage4_pd1 : Delay  DelayLength=6
  Out1 : Outport
  wires:
  In1/1 -> Sum4_stage4/1
  In2/1 -> Sum4_stage4/2
  Sum4_stage4/1 -> Sum4_stage4_pd1/1
  Sum4_stage4_pd1/1 -> Out1/1

== system gm_uz_pmsm_model_6LUT_pd/uz_pmsm_model_6LUT/Sum5 ==
  In1 : Inport
  In2 : Inport  Port=2
  Sum5 : Sum  OutDataTypeStr=single  SampleTime=1e-08
  Sum5_pd1 : Delay  DelayLength=6
  Out1 : Outport
  wires:
  In1/1 -> Sum5/1
  In2/1 -> Sum5/2
  Sum5/1 -> Sum5_pd1/1
  Sum5_pd1/1 -> Out1/1

== system gm_uz_pmsm_model_6LUT_pd/uz_pmsm_model_6LUT/Sum51 ==
  In1 : Inport
  In2 : Inport  Port=2
  Sum51 : Sum  OutDataTypeStr=single  SampleTime=1e-08
  Sum51_pd1 : Delay  DelayLength=6
  Out1 : Outport
  wires:
  In1/1 -> Sum51/1
  In2/1 -> Sum51/2
  Sum51/1 -> Sum51_pd1/1
  Sum51_pd1/1 -> Out1/1

== system gm_uz_pmsm_model_6LUT_pd/uz_pmsm_model_6LUT/Sum52 ==
  In1 : Inport
  In2 : Inport  Port=2
  Sum52 : Sum  OutDataTypeStr=single  SampleTime=1e-08
  Sum52_pd1 : Delay  DelayLength=6
  Out1 : Outport
  wires:
  In1/1 -> Sum52/1
  In2/1 -> Sum52/2
  Sum52/1 -> Sum52_pd1/1
  Sum52_pd1/1 -> Out1/1

== system gm_uz_pmsm_model_6LUT_pd/Current_Controller/Entkopplungen/Lineare_Entkopplung ==
  i_d : Inport
  i_q : Inport  Port=2
  omega_m : Inport  Port=3
  Constant1 : Constant  Value=psi_pm  SampleTime=-1
  Gain : Gain  Gain=L_q
  Gain1 : Gain  Gain=L_d
  Gain2 : Gain  Gain=polepair
  Product : Product
  Product1 : Product
  Sum6 : Sum  Inputs=|++
  u_d : Outport
  u_q : Outport  Port=2
  wires:
  Gain/1 -> Product/1
  Gain2/1 -> Product/2, Product1/2
  Gain1/1 -> Sum6/1
  Product1/1 -> u_q/1
  i_q/1 -> Gain/1
  Constant1/1 -> Sum6/2
  i_d/1 -> Gain1/1
  Product/1 -> u_d/1
  Sum6/1 -> Product1/1
  omega_m/1 -> Gain2/1

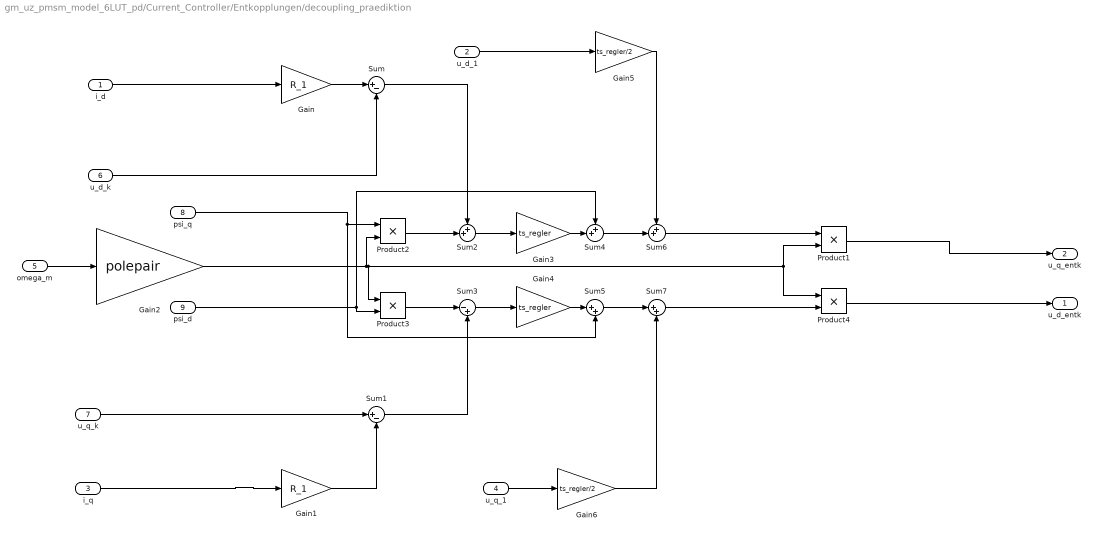
== system gm_uz_pmsm_model_6LUT_pd/Current_Controller/Entkopplungen/decoupling_praediktion ==
  i_d : Inport
  u_d_1 : Inport  Port=2
  i_q : Inport  Port=3
  u_q_1 : Inport  Port=4
  omega_m : Inport  Port=5
  u_d_k : Inport  Port=6
  u_q_k : Inport  Port=7
  psi_q : Inport  Port=8
  psi_d : Inport  Port=9
  Gain : Gain  Gain=R_1
  Gain1 : Gain  Gain=R_1
  Gain2 : Gain  Gain=polepair
  Gain3 : Gain  Gain=ts_regler
  Gain4 : Gain  Gain=ts_regler
  Gain5 : Gain  Gain=ts_regler/2
  Gain6 : Gain  Gain=ts_regler/2
  Product{1..4} (4 alike) : Product
  Sum : Sum  Inputs=|+-
  Sum1 : Sum  Inputs=|+-
  Sum2 : Sum  Inputs=++|
  Sum3 : Sum  Inputs=|-+
  Sum4 : Sum  Inputs=++|
  Sum5 : Sum  Inputs=|++
  Sum6 : Sum  Inputs=++|
  Sum7 : Sum  Inputs=|++
  u_d_entk : Outport
  u_q_entk : Outport  Port=2
  wires:
  Product4/1 -> u_d_entk/1
  Product1/1 -> u_q_entk/1
  i_q/1 -> Gain1/1
  i_d/1 -> Gain/1
  omega_m/1 -> Gain2/1
  Sum7/1 -> Product4/2
  Sum6/1 -> Product1/1
  Gain6/1 -> Sum7/2
  Sum5/1 -> Sum7/1
  Gain5/1 -> Sum6/1
  u_q_1/1 -> Gain6/1
  Sum4/1 -> Sum6/2
  u_d_1/1 -> Gain5/1
  Gain4/1 -> Sum5/1
  Gain3/1 -> Sum4/2
  Sum2/1 -> Gain3/1
  Sum3/1 -> Gain4/1
  Sum1/1 -> Sum3/2
  Sum/1 -> Sum2/1
  Product2/1 -> Sum2/2
  Product3/1 -> Sum3/1
  Gain1/1 -> Sum1/2
  u_q_k/1 -> Sum1/1
  Gain/1 -> Sum/1
  u_d_k/1 -> Sum/2
  Gain2/1 -> Product2/2, Product3/1, Product4/1, Product1/2
  psi_d/1 -> Sum4/1, Product3/2
  psi_q/1 -> Product2/1, Sum5/2

== system gm_uz_pmsm_model_6LUT_pd/Current_Controller/Entkopplungen/static_nonlinear_entkopplung ==
  psi_d : Inport
  psi_q : Inport  Port=2
  omega_m : Inport  Port=3
  Gain2 : Gain  Gain=polepair
  Product : Product
  Product1 : Product
  Scope : Scope  NumInputPorts=2
  u_d : Outport
  u_q : Outport  Port=2
  wires:
  omega_m/1 -> Gain2/1
  psi_d/1 -> Product1/1  "psi_d_LUT"
  Product/1 -> u_d/1, Scope/2
  Product1/1 -> u_q/1, Scope/1
  Gain2/1 -> Product/2, Product1/2
  psi_q/1 -> Product/1  "psi_q_LUT"

== system gm_uz_pmsm_model_6LUT_pd/Current_Controller/Entkopplungen/static_nonlinear_entkopplung1 ==
  psi_d : Inport
  psi_q : Inport  Port=2
  omega_m : Inport  Port=3
  Gain2 : Gain  Gain=polepair
  Product : Product
  Product1 : Product
  Scope : Scope  NumInputPorts=2
  u_d : Outport
  u_q : Outport  Port=2
  wires:
  omega_m/1 -> Gain2/1
  psi_d/1 -> Product1/1  "psi_d_LUT"
  Product/1 -> u_d/1, Scope/2
  Product1/1 -> u_q/1, Scope/1
  Gain2/1 -> Product/2, Product1/2
  psi_q/1 -> Product/1  "psi_q_LUT"
